simulink model "DriveTrain_Modular"  (R2019a)
settings: Solver=VariableStepAuto  StartTime=0.0  StopTime=0.6  RelTol=1e-3
InitFcn:
  | DriveTrainInitialise;
values from neighbouring files (symbols this model uses):
  RotorInertia = 256e3    (= 256000)    [DriveTrainInitialise.m]
libraries: nesl_utility x2, AccumulatorLIB x1, InverterLIB x1, fl_lib x1, MotorLIB x1
settings Model: Creator=plewi  LastModifiedBy=plewi

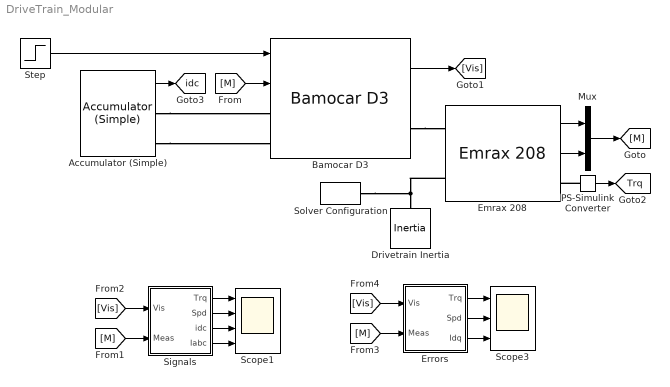
== system DriveTrain_Modular ==
  Accumulator (Simple) : AccumulatorLIB/Accumulator (Simple)  SystemSampleTime=-1
  Bamocar D3 : InverterLIB/Bamocar D3  SystemSampleTime=-1
  Drivetrain Inertia : fl_lib/Mechanical/Rotational Elements/Inertia  inertia=0.01 kg*m^2  w_specify=off  w_priority=High  w=0 rad/s  w_nominal_specify=off  w_nominal_unit=rad/s  w_nominal_value=1  t_specify=off  t_priority=None  t=0 N*m  t_nominal_specify=off  t_nominal_unit=N*m  t_nominal_value=1
  Emrax 208 : MotorLIB/Emrax 208  nPolePairs=PolePairs  pm_flux_linkage=PM  Ld=Ld  Lq=Ld  L0=2e-4  Rs=0.35  J=RotorInertia*1e3
  Errors : Subsystem
  Mux : Mux  Inputs=2
  PS-Simulink Converter : nesl_utility/PS-Simulink Converter  PhysicalDomain=network_engine_domain  SubClassName=ps_output  LeftPortType=input  RightPortType=output  PseudoPeriodic=off  Frequencies=[]  Unit=1  AffineConversion=off
  Scope1 : Scope  NumInputPorts=4
  Scope3 : Scope  NumInputPorts=3
  Signals : Subsystem
  Solver Configuration : nesl_utility/Solver Configuration  PhysicalDomain=network_engine_domain  SubClassName=solver  LeftPortType=input  RightPortType=generic  Tones=[]  Harmonics=[]  SimulateNoise=off  Profile=off  UseLocalSampling=off  EnableSwitchedLinearOptims=on  FrequencyDomain=off  UseCCode=off  RelTol=0.001  AbsTol=1e-06  MinStep=1e-09  ToWorkspace=off  RevertToSquareIcSolve=off  NumHomotopyIterations=100  PhasorMode=off  PhasorModeNumHarmonics=1  DoDC=off  ResidualTolerance=1e-09  UseLocalSolver=off  LocalSolverChoice=NE_BACKWARD_EULER_ADVANCER  LocalSolverSampleTime=0.001  DoFixedCost=off  MaxNonlinIter=3  MaxModeIter=2  LinearAlgebra=auto  EquationFormulation=NE_TIME_EF  DelaysMemoryBudget=1024  AutomaticFiltering=on  FilteringTimeConstant=0.001  PartitionStorageMethod=AS_NEEDED  PartitionMemoryBudget=1024  PartitionMethod=ROBUST
  Step : Step  Time=0.1  After=1000  SampleTime=0
      settings: AttributesFormatString=%<After> at %<Time>s
  tag scope: Trq=global, idc=global
  wires:
  Mux/1 -> [M]
  [M] -> Bamocar D3/2
  Emrax 208/1 -> Mux/1
  Emrax 208/2 -> Mux/2
  Step/1 -> Bamocar D3/1
  Errors/3(Idq) -> Scope3/3
  Errors/1(Trq) -> Scope3/1
  Errors/2(Spd) -> Scope3/2
  Signals/1(Trq) -> Scope1/1
  Signals/2(Spd) -> Scope1/2
  Signals/3(idc) -> Scope1/3
  Signals/4(Iabc) -> Scope1/4
  [M] -> Signals/2("Meas ")
  Bamocar D3/1 -> [Vis]
  PS-Simulink Converter/1 -> [Trq]
  Accumulator (Simple)/1 -> [idc]
  [Vis] -> Signals/1(Vis)
  [Vis] -> Errors/1(Vis)
  [M] -> Errors/2("Meas ")
  connections:
  Bamocar D3/RConn1 -- Emrax 208/LConn1
  Accumulator (Simple)/RConn2 -- Bamocar D3/LConn2
  Emrax 208/LConn2 -- Solver Configuration/RConn1 -- Drivetrain Inertia/LConn1
  PS-Simulink Converter/LConn1 -- Emrax 208/RConn1
  Accumulator (Simple)/RConn1 -- Bamocar D3/LConn1

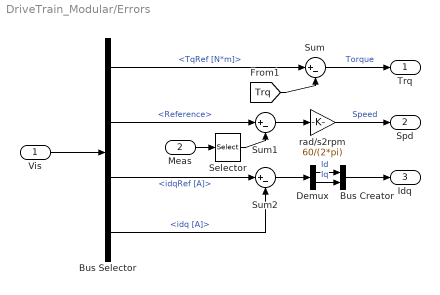
== system DriveTrain_Modular/Errors ==
  Vis : Inport
  "Meas " : Inport  Port=2
  Bus Creator : BusCreator  Inputs=2
  Bus Selector : BusSelector  OutputSignals=TqRef [N*m],Reference,idqRef [A],idq [A]
  Demux : Demux  Outputs=2
  Selector : Selector  InputPortWidth=2  IndexOptions=Index vector (dialog)  Indices=[1]  OutputSizes=1
  Sum : Sum  Inputs=|+-
  Sum1 : Sum  Inputs=|+-
  Sum2 : Sum  Inputs=|+-
  rad/s2rpm : Gain  Gain=60/(2*pi)
  Trq : Outport
  Spd : Outport  Port=2
  Idq : Outport  Port=3
  wires:
  Vis/1 -> Bus Selector/1
  rad/s2rpm/1 -> Spd/1  "Speed"
  Selector/1 -> Sum1/2
  [Trq] -> Sum/2
  Sum1/1 -> rad/s2rpm/1
  Sum/1 -> Trq/1  "Torque"
  Bus Selector/1 -> Sum/1  "<TqRef [N*m]>"
  Bus Selector/3 -> Sum2/1  "<idqRef [A]>"
  Bus Selector/2 -> Sum1/1  "<Reference>"
  "Meas "/1 -> Selector/1
  Bus Selector/4 -> Sum2/2  "<idq [A]>"
  Demux/1 -> Bus Creator/1  "Id"
  Sum2/1 -> Demux/1
  Bus Creator/1 -> Idq/1
  Demux/2 -> Bus Creator/2  "Iq"

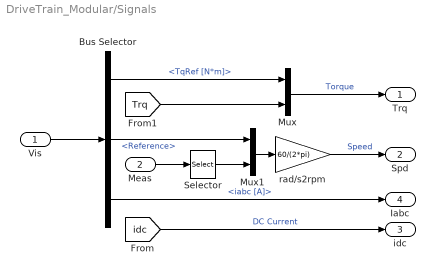
== system DriveTrain_Modular/Signals ==
  Vis : Inport
  "Meas " : Inport  Port=2
  Bus Selector : BusSelector  OutputSignals=TqRef [N*m],Reference,iabc [A]
  Mux : Mux  Inputs=2
  Mux1 : Mux  Inputs=2
  Selector : Selector  InputPortWidth=2  IndexOptions=Index vector (dialog)  Indices=[1]  OutputSizes=1
  rad/s2rpm : Gain  Gain=60/(2*pi)
  Trq : Outport
  Spd : Outport  Port=2
  idc : Outport  Port=3
  Iabc : Outport  Port=4
  wires:
  Vis/1 -> Bus Selector/1
  rad/s2rpm/1 -> Spd/1  "Speed"
  Selector/1 -> Mux1/2
  [Trq] -> Mux/2
  Mux1/1 -> rad/s2rpm/1
  [idc] -> idc/1  "DC Current"
  Mux/1 -> Trq/1  "Torque"
  Bus Selector/1 -> Mux/1  "<TqRef [N*m]>"
  Bus Selector/3 -> Iabc/1  "<iabc [A]>"
  Bus Selector/2 -> Mux1/1  "<Reference>"
  "Meas "/1 -> Selector/1
